simulink model "metodoM1"  (R2012b)
settings: Solver=ode45  StartTime=0.0  StopTime=1  RelTol=1e-3
libraries: Encoder x2, BLDC x1
settings Model: Creator=h3now  LastModifiedBy=h3now

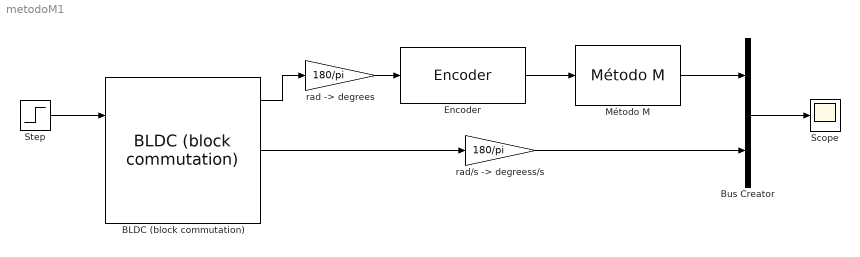
== system metodoM1 ==
  BLDC (block commutation) : BLDC/BLDC (block commutation)  J=1.39e-6  R=10.1/2  L=2.04/2000  P=8  Kt=15.7e-3/1.19  Ke=15.7e-3/1.19  Kd=0
  Bus Creator : BusCreator  Inputs=2
  Encoder : Encoder/Encoder  Nr=360
  Método M : Encoder/Método M  Ts=0.05
  Scope : Scope
      settings: YMin=12500  YMax=45000
  Step : Step  Time=0.31  Before=12  After=0  SampleTime=0
  "rad -> degrees" : Gain  Gain=180/pi
  "rad/s -> degreess/s" : Gain  Gain=180/pi
  wires:
  Step/1 -> BLDC (block commutation)/1
  BLDC (block commutation)/2 -> "rad/s -> degreess/s"/1
  Bus Creator/1 -> Scope/1
  "rad/s -> degreess/s"/1 -> Bus Creator/2
  Encoder/1 -> Método M/1
  Método M/1 -> Bus Creator/1
  BLDC (block commutation)/1 -> "rad -> degrees"/1
  "rad -> degrees"/1 -> Encoder/1
